simulink model "blade"  (Simulink 7.7)
settings: Solver=ode45  StartTime=T_init  StopTime=T_limit  RelTol=1e-3
values from neighbouring files (symbols this model uses):
  Bpb = Bpb*sum(Cpb)    [bladeData.m]
  Bpb2 = Bpb2*sum(Cpb2)    [bladeData.m]
  Constant_Beta_1_m1 = 5    [bladeData.m]
  Cpb = Cpb/sum(Cpb)    [bladeData.m]
  Cpb2 = Cpb2/sum(Cpb2)    [bladeData.m]
  Gain_Beta_2_m2 = 1.2    [bladeData.m]
  seed = randi(10^6,[1,2])    [bladeData.m]
  Ts = 0.01    [bladeData.m]    (also in msfcn_ff.m = block.DialogPrm(2).Data; run.m)
undefined symbols (not defined in the file or in its folder): Apb, Apb2
libraries: simulink x4
settings Model: Creator=pcasau  LastModifiedBy=pcasau
settings DataIOCC: SignalLoggingSaveFormat=Dataset
settings OptimizationCC: ExpressionDepthLimit=128
settings DebuggingCC: FcnCallInpInsideContextMsg=Enable All
settings CodeAppCC: CustomSymbolStrType=$N$R$M_T
settings GRTTargetCC: CombineOutputUpdateFcns=on

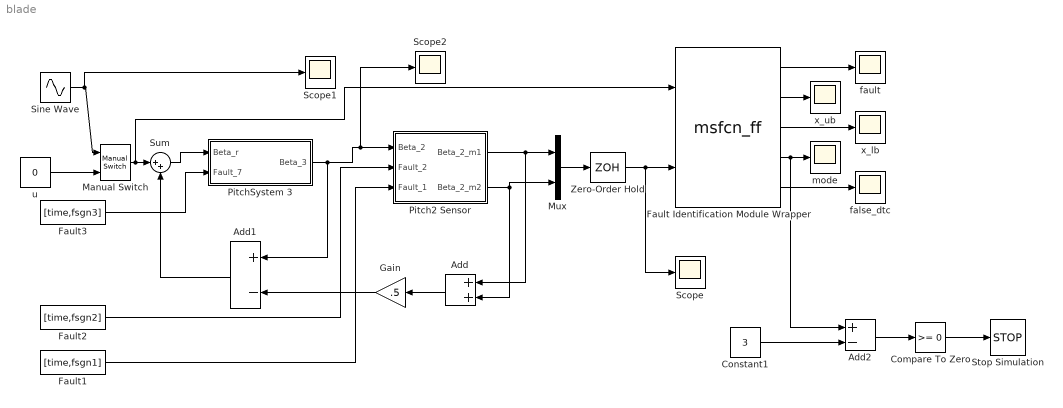
== system blade ==
  Add : Sum
  Add1 : Sum  Inputs=+-
  Add2 : Sum  Inputs=+-
  Compare To Zero : simulink/Logic and Bit Operations/Compare To Zero  SystemSampleTime=-1  relop=>=  LogicOutDataTypeMode=boolean
  Constant1 : Constant  Value=3
  Fault Identification Module Wrapper : M-S-Function  FunctionName=msfcn_ff  Parameters=ff, Ts, Ad, Bd, Ld, Cd, Dd, Nd, wp, wm, A3, B3, L3, C3, D3, N3,wp3, wm3, Aglb, Bglb, Lglb, Cglb, Dglb, Nglb, A2, B2, L2, C2, D2, N2, wp2, wm2, A1, B1, L1, C1, D1, N1, wp1, wm1
  Fault1 : FromWorkspace  VariableName=[time,fsgn1]  SampleTime=Ts
  Fault2 : FromWorkspace  VariableName=[time,fsgn2]  SampleTime=Ts
  Fault3 : FromWorkspace  VariableName=[time,fsgn3]  SampleTime=Ts
  Gain : Gain  Gain=.5
  Manual Switch : simulink/Signal Routing/Manual Switch  SystemSampleTime=-1  sw=1  action=0  varsize=off
  Mux : Mux  Inputs=2
  Pitch2 Sensor : Subsystem
  PitchSystem 3 : Subsystem
  Scope : Scope
      settings: SaveName=beta_m  DataFormat=Array  SampleInput=on  SampleTime=Ts
  Scope1 : Scope
      settings: SaveName=u  DataFormat=Array  SampleInput=on  SampleTime=Ts
  Scope2 : Scope
      settings: SaveName=beta  DataFormat=Array  SampleInput=on  SampleTime=Ts
  Sine Wave : Sin  SineType=Sample based  Amplitude=8  Samples=105  SampleTime=Ts
  Stop Simulation : Stop
  Sum : Sum  Inputs=|++
  Zero-Order Hold : ZeroOrderHold  SampleTime=Ts
  false_dtc : Scope
      settings: YMin=-1  YMax=1  SaveName=false_dtc  DataFormat=Array  SampleInput=on  SampleTime=Ts
  fault : Scope
      settings: YMin=0.95  YMax=1.05  SaveName=fault  DataFormat=Array  SampleInput=on  SampleTime=Ts
  mode : Scope
      settings: YMin=-1  YMax=1  SaveName=mode  DataFormat=Array  SampleInput=on  SampleTime=Ts
  u : Constant  Value=0
  x_lb : Scope
      settings: YMin=-1  YMax=1  SaveName=x_lb  DataFormat=Array  SampleInput=on  SampleTime=Ts
  x_ub : Scope
      settings: YMin=-1  YMax=1  SaveName=x_ub  DataFormat=Array  SampleInput=on  SampleTime=Ts
  wires:
  Fault Identification Module Wrapper/1 -> fault/1
  Fault Identification Module Wrapper/2 -> x_ub/1
  Fault Identification Module Wrapper/3 -> x_lb/1
  Fault Identification Module Wrapper/5 -> false_dtc/1
  PitchSystem 3/1(Beta_3) -> Add1/1, Pitch2 Sensor/1(Beta_2), Scope2/1
  Pitch2 Sensor/1(Beta_2_m1) -> Add/1, Mux/1
  Pitch2 Sensor/2(Beta_2_m2) -> Mux/2, Add/2
  Add/1 -> Gain/1
  Add1/1 -> Sum/2
  Gain/1 -> Add1/2
  Mux/1 -> Zero-Order Hold/1
  Zero-Order Hold/1 -> Scope/1, Fault Identification Module Wrapper/2
  Sum/1 -> PitchSystem 3/1(Beta_r)
  Fault Identification Module Wrapper/4 -> Add2/1, mode/1
  Add2/1 -> Compare To Zero/1
  Constant1/1 -> Add2/2
  Compare To Zero/1 -> Stop Simulation/1
  Sine Wave/1 -> Scope1/1, Manual Switch/1
  u/1 -> Manual Switch/2
  Manual Switch/1 -> Fault Identification Module Wrapper/1, Sum/1
  Fault3/1 -> PitchSystem 3/2(Fault_7)
  Fault2/1 -> Pitch2 Sensor/2(Fault_2)
  Fault1/1 -> Pitch2 Sensor/3(Fault_1)

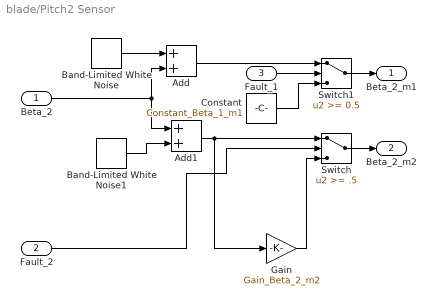
== system blade/Pitch2 Sensor ==
  Beta_2 : Inport
  Fault_2 : Inport  Port=2
  Fault_1 : Inport  Port=3
  Add : Sum
  Add1 : Sum
  Band-Limited White Noise : simulink/Sources/Band-Limited White Noise  SystemSampleTime=-1  Cov=Np_beta  Ts=Ts  seed=seed(1)
  Band-Limited White Noise1 : simulink/Sources/Band-Limited White Noise  SystemSampleTime=-1  Cov=Np_beta  Ts=Ts  seed=seed(2)
  Constant : Constant  Value=Constant_Beta_1_m1
  Gain : Gain  Gain=Gain_Beta_2_m2
  Switch : Switch  Threshold=.5
  Switch1 : Switch  Threshold=0.5
  Beta_2_m1 : Outport
  Beta_2_m2 : Outport  Port=2
  wires:
  Band-Limited White Noise1/1 -> Add1/2
  Band-Limited White Noise/1 -> Add/1
  Beta_2/1 -> Add1/1, Add/2
  Add1/1 -> Gain/1, Switch/1
  Gain/1 -> Switch/3
  Switch/1 -> Beta_2_m2/1
  Fault_2/1 -> Switch/2
  Add/1 -> Switch1/1
  Fault_1/1 -> Switch1/2
  Constant/1 -> Switch1/3
  Switch1/1 -> Beta_2_m1/1

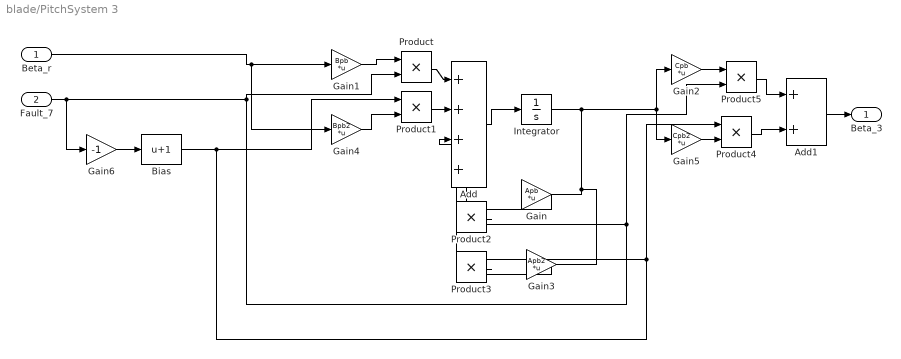
== system blade/PitchSystem 3 ==
  Beta_r : Inport
  Fault_7 : Inport  Port=2
  Add : Sum  Inputs=++++
  Add1 : Sum
  Bias : Bias  Bias=1
  Gain : Gain  Gain=Apb  Multiplication=Matrix(K*u)
  Gain1 : Gain  Gain=Bpb  Multiplication=Matrix(K*u)
  Gain2 : Gain  Gain=Cpb  Multiplication=Matrix(K*u)
  Gain3 : Gain  Gain=Apb2  Multiplication=Matrix(K*u)
  Gain4 : Gain  Gain=Bpb2  Multiplication=Matrix(K*u)
  Gain5 : Gain  Gain=Cpb2  Multiplication=Matrix(K*u)
  Gain6 : Gain  Gain=-1
  Integrator : Integrator
  Product{,1..5} (6 alike) : Product  RndMeth=Zero
  Beta_3 : Outport
  wires:
  Beta_r/1 -> Gain4/1, Gain1/1
  Fault_7/1 -> Product2/2, Product5/2, Product/2, Gain6/1
  Gain4/1 -> Product1/2
  Add/1 -> Integrator/1
  Integrator/1 -> Gain5/1, Gain2/1, Gain3/1, Gain/1
  Product/1 -> Add/1
  Gain1/1 -> Product/1
  Product1/1 -> Add/2
  Gain3/1 -> Product3/2
  Gain/1 -> Product2/1
  Product2/1 -> Add/4
  Product3/1 -> Add/3
  Add1/1 -> Beta_3/1
  Gain2/1 -> Product5/1
  Gain5/1 -> Product4/2
  Product4/1 -> Add1/2
  Product5/1 -> Add1/1
  Gain6/1 -> Bias/1
  Bias/1 -> Product1/1, Product3/1, Product4/1
